simulink library "PI_Lib"  (R2020b)
settings: Solver=VariableStepAuto  StartTime=0.0  StopTime=10.0  RelTol=1e-3
settings Model: Creator=vijay jagtap  LastModifiedBy=vijay jagtap

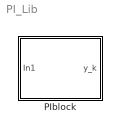
== system PI_Lib ==
  PIblock : Subsystem  mask{Kp=35, Ki=600, Ts=0.01}
      mask Display: image('download.jpg'); % Use "Edit Image" on toolstrip to change.

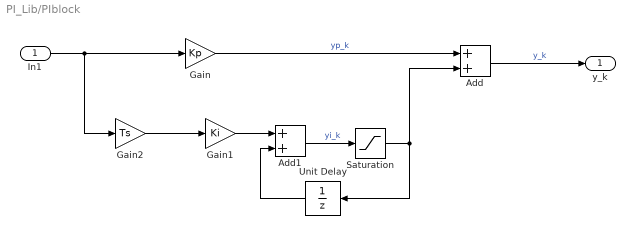
== system PI_Lib/PIblock ==
  In1 : Inport
  Add : Sum
  Add1 : Sum
  Gain : Gain  Gain=Kp
  Gain1 : Gain  Gain=Ki
  Gain2 : Gain  Gain=Ts
  Saturation : Saturate  UpperLimit=1  LowerLimit=-1
  Unit Delay : UnitDelay  SampleTime=-1  HasFrameUpgradeWarning=on
  y_k : Outport
  wires:
  Saturation/1 -> Add/2, Unit Delay/1
  Gain/1 -> Add/1  "yp_k"
  Add/1 -> y_k/1  "y_k"
  Add1/1 -> Saturation/1  "yi_k"
  Unit Delay/1 -> Add1/2
  In1/1 -> Gain2/1, Gain/1
  Gain1/1 -> Add1/1
  Gain2/1 -> Gain1/1
